simulink model "system_model"  (R2022b)
settings: Solver=VariableStepAuto  StartTime=0.0  StopTime=10.0  RelTol=1e-3
values from neighbouring files (symbols this model uses):
  DT = 5    [load_ECM_params.m]    (also in load_params.m)
  param = CellParametersFunction_MC_modstudy(param)    [load_params.m]
libraries: simulink x2, sharedTrackingLibrary x1
settings Model: Creator=adamp  LastModifiedBy=adamp
settings SolverCC: AlgebraicLoopSolver=TrustRegion
settings DataIOCC: ExternalInput=param, param  LoadExternalInput=on
settings DebuggingCC: UnconnectedInputMsg=warning  UnconnectedOutputMsg=warning  UnconnectedLineMsg=warning  SFMachineParentedDataDiag=warning
settings ModelReferenceCC: EnableRefExpFcnMdlSchedulingChecks=on

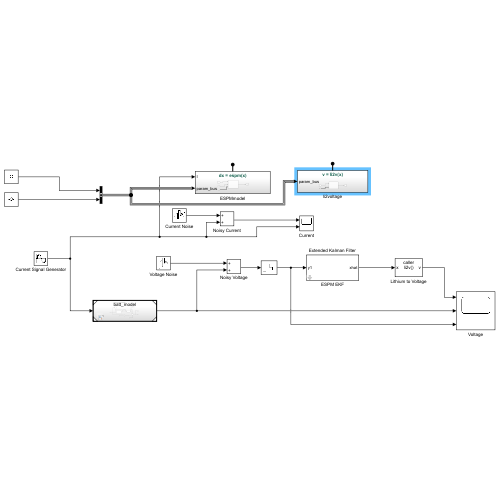
[thumbnail: Simulink's stored preview of the top-level diagram]
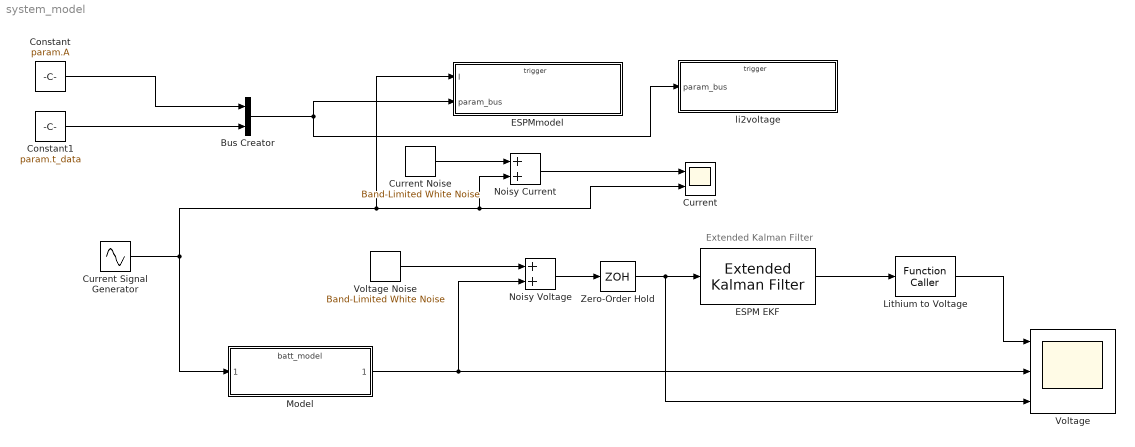
== system system_model ==
  note: Extended Kalman Filter
  Bus Creator : BusCreator  Inputs=2
  Constant : Constant  Value=param.A
  Constant1 : Constant  Value=param.t_data
  Current : Scope  NumInputPorts=2
  Current Noise : simulink/Sources/Band-Limited White Noise  Cov=[0.005]  Ts=DT  seed=[23341]
  Current Signal Generator : Sin  SampleTime=DT
  ESPM EKF : sharedTrackingLibrary/Extended Kalman Filter  StateTransitionFcn=espm  HasStateTransitionJacobianFcn=off  HasAdditiveProcessNoise=Additive  ProcessNoise=1  HasTimeVaryingProcessNoise=off  HasStateTransitionFcnExtraArgument=0  InitialState=x_initial  InitialStateCovariance=1  MeasurementFcn1=li2v  HasMeasurementJacobianFcn1=off  HasMeasurementEnablePort1=off  HasAdditiveMeasurementNoise1=Additive  MeasurementNoise1=1  HasTimeVaryingMeasurementNoise1=off  HasMeasurementFcnExtraArgument1=0  HasMeasurementWrapping1=off  MeasurementFcn2=myMeasurementFcn  HasMeasurementJacobianFcn2=off  HasMeasurementEnablePort2=off  HasAdditiveMeasurementNoise2=Additive  MeasurementNoise2=1  HasTimeVaryingMeasurementNoise2=off  HasMeasurementFcnExtraArgument2=0  HasMeasurementWrapping2=off  MeasurementFcn3=myMeasurementFcn  HasMeasurementJacobianFcn3=off  HasMeasurementEnablePort3=off  HasAdditiveMeasurementNoise3=Additive  MeasurementNoise3=1  HasTimeVaryingMeasurementNoise3=off  HasMeasurementFcnExtraArgument3=0  HasMeasurementWrapping3=off  MeasurementFcn4=myMeasurementFcn  HasMeasurementJacobianFcn4=off  HasMeasurementEnablePort4=off  HasAdditiveMeasurementNoise4=Additive  MeasurementNoise4=1  HasTimeVaryingMeasurementNoise4=off  HasMeasurementFcnExtraArgument4=0  HasMeasurementWrapping4=off  MeasurementFcn5=myMeasurementFcn  HasMeasurementJacobianFcn5=off  HasMeasurementEnablePort5=off  HasAdditiveMeasurementNoise5=Additive  MeasurementNoise5=1  HasTimeVaryingMeasurementNoise5=off  HasMeasurementFcnExtraArgument5=0  HasMeasurementWrapping5=off  EnableMultirate=off  StateTransitionFcnSampleTime=1  MeasurementFcn1SampleTime=1  MeasurementFcn2SampleTime=1  MeasurementFcn3SampleTime=1  MeasurementFcn4SampleTime=1  MeasurementFcn5SampleTime=1  UseCurrentEstimator=on  OutputStateCovariance=off  DataType=double  SampleTime=DT  NumberOfMeasurements=1
  ESPMmodel : Subsystem  TreatAsAtomicUnit=on
  Lithium to Voltage : FunctionCaller  FunctionPrototype=v = li2v(x)  InputArgumentSpecifications=<Enter example>  OutputArgumentSpecifications=<Enter example>
  Model : ModelReference  ModelNameDialog=batt_model.slx  SimulationMode=Normal  ModelReferenceVersion=6.18
  Noisy Current : Sum
  Noisy Voltage : Sum
  Voltage : Scope  NumInputPorts=3
  Voltage Noise : simulink/Sources/Band-Limited White Noise  Cov=[0.02]  Ts=DT  seed=[23341]
  Zero-Order Hold : ZeroOrderHold  SampleTime=DT
  li2voltage : Subsystem  TreatAsAtomicUnit=on
  wires:
  Current Signal Generator/1 -> Model/1, ESPMmodel/1(I), Current/2, Noisy Current/2
  Model/1 -> Noisy Voltage/2, Voltage/2
  Voltage Noise/1 -> Noisy Voltage/1
  Current Noise/1 -> Noisy Current/1
  Noisy Current/1 -> Current/1
  Noisy Voltage/1 -> Zero-Order Hold/1
  ESPM EKF/1 -> Lithium to Voltage/1
  Lithium to Voltage/1 -> Voltage/1
  Zero-Order Hold/1 -> ESPM EKF/1, Voltage/3
  Constant/1 -> Bus Creator/1
  Constant1/1 -> Bus Creator/2
  Bus Creator/1 -> ESPMmodel/2(param_bus), li2voltage/1(param_bus)

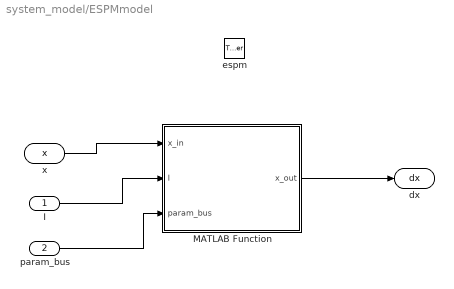
== system system_model/ESPMmodel ==
  I : Inport
  param_bus : Inport  Port=2
  espm : TriggerPort  TriggerType=function-call  IsSimulinkFunction=on  FunctionName=espm  FunctionVisibility=scoped  VariantControl=(inherit)
  MATLAB Function : MATLAB Function  TreatAsAtomicUnit=on
  x : ArgIn  DisableCoverage=on  PortDimensions=n_states  ArgumentName=x
  dx : ArgOut  DisableCoverage=on  PortDimensions=n_states  ArgumentName=dx
  wires:
  x/1 -> MATLAB Function/1(x_in)
  MATLAB Function/1(x_out) -> dx/1
  I/1 -> MATLAB Function/2(I)
  param_bus/1 -> MATLAB Function/3(param_bus)

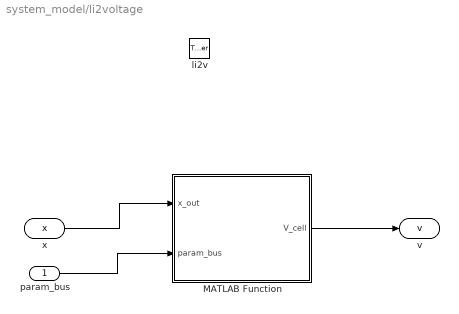
== system system_model/li2voltage ==
  param_bus : Inport
  li2v : TriggerPort  TriggerType=function-call  IsSimulinkFunction=on  FunctionName=li2v  FunctionVisibility=scoped  VariantControl=(inherit)
  MATLAB Function : MATLAB Function  TreatAsAtomicUnit=on
  x : ArgIn  DisableCoverage=on  PortDimensions=n_states  ArgumentName=x
  v : ArgOut  DisableCoverage=on  ArgumentName=v
  wires:
  x/1 -> MATLAB Function/1(x_out)
  MATLAB Function/1(V_cell) -> v/1
  param_bus/1 -> MATLAB Function/2(param_bus)

== matlab function system_model/ESPMmodel/MATLAB Function ==
  data: x_in input size=n_states; x_out output size=n_states; I input size=1; param_bus input
function x_out = ESPMmodel(x_in, I, param_bus)  % param
param = param_bus;
% applied current = Nc*nominal current value
I_multiply = I;
param.I_data = I_multiply*ones(length(param.t_data),1); % current vector

%I_cell_prev = param.I_data(1)/param.Nc*ones(param.Nc,1);

tspan = param.t_data;

%% Solve ODEs 
reltol=5.0e-09; abstol=5.0e-09;
event_formatted = @(t,x) physical_event_function(t,x,param); 
options=odeset('RelTol',reltol,'AbsTol',abstol,'Events',event_formatted);
[t_out, x_out,te,xe,ie] = ode15s(@(t_out, x_out) Cell_ode(t_out, x_out, param), tspan, x_in, options);

%Transpose state matrix into row form to match established data structure 
x_out = real(x_out'); %Keep the result real

== matlab function system_model/li2voltage/MATLAB Function ==
  data: x_out input size=n_states; V_cell output size=1; param_bus input
function V_cell =li2voltage(x_out, param_bus)
param = param_bus;
%% Separate electrochemical, thermal & aging state variables from x_out matrix
%Define solid concentrations
cs = x_out(1:(param.Nr-1)*param.Nc*2,:);            %All solid concentrations
cs_n = cs(1:(param.Nr-1)*param.Nc,:);               %Anode Concentrations
cs_p = cs((param.Nr-1)*param.Nc+1:end,:);           %Cathode Concentrations

index_cs = (param.Nr-1)*param.Nc*2;                 %Index for final solid concentration
index_ce = index_cs + param.Nc*param.ce_states;     %Index for final electrolyte concentration

%Define electrolyte concentrations
ce = x_out(index_cs+1:index_ce,:);                  %All electrolyte concentrations
ce_n = ce(1:param.Nx_n*param.Nc,:);                 %Negative Electrolyte Region
ce_s = ce(param.Nx_n*param.Nc+1:(param.Nx_n + param.Nx_s)*param.Nc,:); %Separator Region
ce_p = ce((param.Nx_n + param.Nx_s)*param.Nc+1:param.ce_states*param.Nc,:); %Positive Region

%% Temperature dependent transport and kinetics for each cell

for j = 1:length(cs(1,:))
    I_cell(1,j) = param.I_data(j);  
    T_core(1,j) = param.T_amb;
    T_surf(1,j) = param.T_amb;
    % Surface concentration -> surface stoichiometry
    for i = 1:param.Nc
        theta_surf_n(i,j) = cs_n(i*(param.Nr-1),j)/param.c_n_max;
        theta_surf_p(i,j) = cs_p(i*(param.Nr-1),j)/param.c_p_max;
    end
    
    % Temperature dependence
    [Dsn(:,j), Dsp(:,j), kn(:,j), kp(:,j)] = arrhenius_temp(param, T_core(:,j));

    
    % Define electrolyte boundary concentrations for each cell
    for i = 1:param.Nc
        index1n = (i-1)*param.Nx_n+1;
        index2n = i*param.Nx_n;
        index1s = (i-1)*param.Nx_s+1;
        index2s = i*param.Nx_s;
        index1p = (i-1)*param.Nx_p+1;
        index2p = i*param.Nx_p;
      
        %Average Electrolyte Concentrations for conc. dependent parameters
        ce_n_avg(i,j) = mean(ce_n(index1n:index2n,j));
        ce_s_avg(i,j) = mean(ce_s(index1s:index2s,j));
        ce_p_avg(i,j) = mean(ce_p(index1p:index2p,j));
        %ce_all(Row = 'Grid point', Column = 'Time point', 3rd Dimension = 'Cell #')
        ce_all(:,j,i) = [ce_n(index1n:index2n,j); ce_s(index1s:index2s,j); ce_p(index1p:index2p,j)];
        
        %ce_all_avg(Row = 'Cell #', Column = 'Time point')
        ce_all_avg(i,j) = mean(ce_all(:,j,i));
        
    end
    eps_el_n = param.eps_el_n_ref;
    % Electrolyte Conductivity
    [K_el_eff_n(:,j),K_el_eff_s(:,j),K_el_eff_p(:,j)] = conductivity_update(ce_n_avg(:,j)...
        ,ce_s_avg(:,j),ce_p_avg(:,j),eps_el_n,T_core(:,j),param);
    
    % Open circuit potential and overpotential
    ocp_p(:,j) = U_p(theta_surf_p(:,j));
    ocp_n(:,j) = U_n(theta_surf_n(:,j));
    
   
    % NOTE TO SELF: replace all param.I_data with I_cell
    % Using I_cell, update current-dependent electrochemical parameters
    eta_p(:,j) = eta_cathode(theta_surf_p(:,j), ce_p_avg(:,j), T_core(:,j), I_cell(:,j), param, kp(:,j));
    eta_n(:,j) = eta_anode(theta_surf_n(:,j), ce_n_avg(:,j), T_core(:,j), I_cell(:,j), param, kn(:,j));


    % Cell voltages
    [phi_e(:,j),R_el(:,j)] = electrolyte_potential(ce_all_avg(:,j), ce_all(:,j,:),K_el_eff_n(:,j),...
        K_el_eff_s(:,j), K_el_eff_p(:,j),T_core(:,j), I_cell(:,j), param);
    V_cell(:,j) = V_calculation(ocp_p(:,j),ocp_n(:,j),eta_p(:,j),eta_n(:,j),...
        phi_e(:,j),I_cell(:,j),param);
    V_oc = ocp_p - ocp_n;
end


%% Calculate SOC
%[soc_bulk_n,soc_bulk_p] = soc_calculation(cs_n,cs_p,param);
